simulink library "MinSegLibrary_M2V3"  (R2015a)
settings: Solver=ode45  StartTime=0.0  StopTime=10.0  RelTol=1e-3
libraries: arduinolib x4, simulink x2
settings Model: Creator=hurstj  LastModifiedBy=hurstj
settings DebuggingCC: UnderspecifiedInitializationDetection=Classic  MergeDetectMultiDrivingBlocksExec=none  SolverPrmCheckMsg=warning  StateNameClashWarn=warning

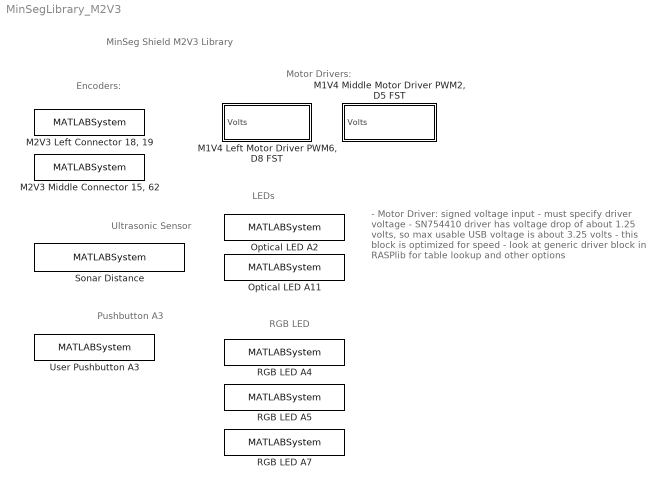
== system MinSegLibrary_M2V3 ==
  note: MinSeg Shield M2V3 Library
  note: Motor Drivers:
  note: Ultrasonic Sensor
  note: Encoders:
  note: RGB LED
  note: Pushbutton A3
  note: LEDs
  note: - Motor Driver: signed voltage input
      | - must specify driver voltage
      | - SN754410 driver has voltage drop of about 1.25 volts, so max usable USB voltage is about 3.25 volts
      | - this block is optimized for speed
      | - look at generic driver block in RASPlib for table lookup and other options
  "M1V4 Left Motor Driver PWM6, D8 FST" : Subsystem  mask{Vsupply=3.25}
      mask prompts: Vsupply "Driver Voltage"
      mask help: Specify driver supply voltage (3.25 for USB with SN75441)
      mask Display:
      | port_label('input',1,'Volts')
      | text(15,5,['Vsupply=' num2str(Vsupply)])
  "M1V4 Middle Motor Driver PWM2, D5 FST" : Subsystem  mask{Vsupply=3.25}
      mask prompts: Vsupply "Driver Voltage"
      mask help: Specify driver supply voltage (3.25 for USB with SN75441)
      mask Display:
      | port_label('input',1,'Volts')
      | text(15,5,['Vsupply=' num2str(Vsupply)])
  "M2V3 Left Connector 18, 19" : MATLABSystem  System=Encoder_arduino  Encoder=1  PinA=19  PinB=18  PWMFSelect=3  PWMTimer=-1
      mask Type: Encoder_arduino
      mask Display:
      | disp('soEncoder');
      | port_label('output',1,'y');
  "M2V3 Middle Connector 15, 62" : MATLABSystem  System=Encoder_arduino  Encoder=3  PinA=15  PinB=62  PWMFSelect=3  PWMTimer=-1
      mask Type: Encoder_arduino
      mask Display:
      | disp('soEncoder');
      | port_label('output',1,'y');
  Optical LED A11 : MATLABSystem  System=soDAnalogWrite  Pin=11
      mask Type: soDAnalogWrite
      mask Display:
      | disp('Analog Digital Write');
      | port_label('input',1,'u');
  Optical LED A2 : MATLABSystem  System=soDAnalogWrite  Pin=2
      mask Type: soDAnalogWrite
      mask Display:
      | disp('Analog Digital Write');
      | port_label('input',1,'u');
  RGB LED A4 : MATLABSystem  System=soDAnalogWrite  Pin=4
      mask Type: soDAnalogWrite
      mask Display:
      | disp('Analog Digital Write');
      | port_label('input',1,'u');
  RGB LED A5 : MATLABSystem  System=soDAnalogWrite  Pin=5
      mask Type: soDAnalogWrite
      mask Display:
      | disp('Analog Digital Write');
      | port_label('input',1,'u');
  "RGB LED A7 " : MATLABSystem  System=soDAnalogWrite  Pin=7
      mask Type: soDAnalogWrite
      mask Display:
      | disp('Analog Digital Write');
      | port_label('input',1,'u');
  Sonar Distance : MATLABSystem  System=soHCSR04Sonar  TrigPin=12  EchoPin=11
      mask Type: soHCSR04Sonar
      mask Display:
      | disp('soHCSR04Sonar');
      | port_label('output',1,'d_cm');
  User Pushbutton A3 : MATLABSystem  System=soDAnalogRead  Pin=3
      mask Type: soDAnalogRead
      mask Display:
      | disp('Analog Digital Read');
      | port_label('output',1,'y');

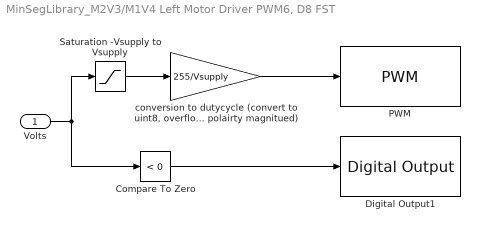
== system MinSegLibrary_M2V3/M1V4 Left Motor Driver PWM6, D8 FST ==
  Volts : Inport
  Compare To Zero : simulink/Logic and Bit Operations/Compare To Zero  relop=<  OutDataTypeStr=boolean
  Digital Output1 : arduinolib/Digital Output  pinNumber=8  blockPlatform=arduino
  PWM : arduinolib/PWM  pinNumber=6  blockPlatform=arduino
  Saturation -Vsupply to Vsupply : Saturate  UpperLimit=Vsupply  LowerLimit=-Vsupply  OutDataTypeStr=single
  "conversion to dutycycle (convert to uint8, overflow will provide reverse polairty magnitued)" : Gain  Gain=255/Vsupply  OutDataTypeStr=uint8
  wires:
  Volts/1 -> Compare To Zero/1, Saturation -Vsupply to Vsupply/1
  Saturation -Vsupply to Vsupply/1 -> "conversion to dutycycle (convert to uint8, overflow will provide reverse polairty magnitued)"/1
  "conversion to dutycycle (convert to uint8, overflow will provide reverse polairty magnitued)"/1 -> PWM/1
  Compare To Zero/1 -> Digital Output1/1

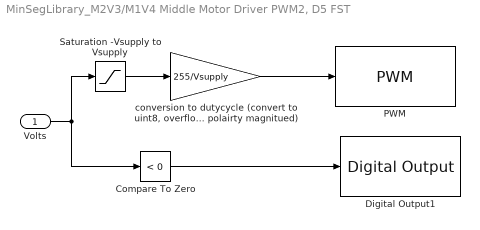
== system MinSegLibrary_M2V3/M1V4 Middle Motor Driver PWM2, D5 FST ==
  Volts : Inport
  Compare To Zero : simulink/Logic and Bit Operations/Compare To Zero  relop=<  OutDataTypeStr=boolean
  Digital Output1 : arduinolib/Digital Output  pinNumber=5  blockPlatform=arduino
  PWM : arduinolib/PWM  pinNumber=2  blockPlatform=arduino
  Saturation -Vsupply to Vsupply : Saturate  UpperLimit=Vsupply  LowerLimit=-Vsupply  OutDataTypeStr=single
  "conversion to dutycycle (convert to uint8, overflow will provide reverse polairty magnitued)" : Gain  Gain=255/Vsupply  OutDataTypeStr=uint8
  wires:
  Compare To Zero/1 -> Digital Output1/1
  "conversion to dutycycle (convert to uint8, overflow will provide reverse polairty magnitued)"/1 -> PWM/1
  Saturation -Vsupply to Vsupply/1 -> "conversion to dutycycle (convert to uint8, overflow will provide reverse polairty magnitued)"/1
  Volts/1 -> Saturation -Vsupply to Vsupply/1, Compare To Zero/1
